simulink model "MATLAB_TEST"  (R2019b)
settings: Solver=FixedStepDiscrete  StartTime=0  StopTime=50  FixedStep=0.0025  RelTol=1e-3
undefined symbols (not defined in the file): BCM_COM_PROC_P20, BCM_COM_PROC_P20_SFW_R2018b, BCM_COM_PROC_P2_5, BCM_COM_PROC_P2_5_SFW_R2018b, BCM_COM_PROC_P5, BCM_COM_PROC_P5_SFW_R2018b, BCMA_ACCU_PT_Conf_Flt, BCMA_ACCU_PT_Unconf_Flt, BCMA_Antiskid_Off_Sanction, BCMA_Avionics_Conf_Flt, BCMA_BCM_CCDL_Conf_Flt, BCMA_BCM_CCDL_Unconf_Flt, BCMA_BCM_DBCU_INHIBITION_Conf_Flt, BCMA_BCM_DBCU_INHIBITION_Unconf_Flt, BCMA_BCP_ALT_Disp_Sw_Conf_Flt, BCMA_BCP_ALT_Disp_Sw_Unconf_Flt, BCMA_BCP_ALT_SW_ON_CMD_Conf_Flt, BCMA_BCP_ALT_SW_ON_CMD_Unconf_Flt, BCMA_BCP_PARK_OFF_SW_CMD_Conf_Flt, BCMA_BCP_PARK_OFF_SW_CMD_Unconf_Flt, BCMA_CF_BSELV_JCL, BCMA_CF_BSELV_JOP, BCMA_CF_BSELV_OC, BCMA_CF_BSELV_SC, BCMA_CF_LH_SV_JCL, BCMA_CF_LH_SV_JOP, BCMA_CF_LH_SV_OC, BCMA_CF_LH_SV_SC, BCMA_CF_PARK_BRK, BCMA_CF_RESIDUAL_PRESS, BCMA_CF_RH_SV_JCL, BCMA_CF_RH_SV_JOP, BCMA_CF_RH_SV_OC, BCMA_CF_RH_SV_SC, BCMA_CF_SELV_JCL, BCMA_CF_SELV_JOP, BCMA_CF_SELV_OC, BCMA_CF_SELV_SC, BCMA_CF_SV_DRIFT, BCMA_DBCU_ALT_MODE_Conf_Flt, BCMA_DBCU_ALT_MODE_Unconf_Flt, BCMA_DBCU_BRK_ORDER_FAIL_Conf_Flt, BCMA_DBCU_BRK_ORDER_FAIL_Unconf_Flt, BCMA_DBCU_Conf_Flt, BCMA_DBCU_DISPATCH_SW_ON_Conf_Flt, BCMA_DBCU_DISPATCH_SW_ON_Unconf_Flt, BCMA_DBCU_FAILED_Conf_Flt, BCMA_DBCU_FAILED_Unconf_Flt, BCMA_DFCS1_Capsule_Validity, BCMA_DFCS1_Label202_Corrupted, BCMA_DFCS1_Label202_Not_Refreshed, BCMA_DFCS1_Label204_Corrupted, BCMA_DFCS1_Label204_Not_Refreshed, BCMA_DFCS1_Label205_Corrupted, BCMA_DFCS1_Label205_Not_Refreshed, BCMA_DFCS1_Label206_Corrupted, BCMA_DFCS1_Label206_Not_Refreshed, BCMA_DFCS1_Label207_Corrupted, BCMA_DFCS1_Label207_Not_Refreshed, BCMA_DFCS3_Capsule_Validity ... (+762)
libraries: simulink x73, lib_MBD_Control x5
(part 9 of 16)

== system MATLAB_TEST/AVIONICS/Brake_Control_Module_Side_A/BCSA Controller CP/DFCSB_Label202_Validity1 ==
  Capsule_Validity : Inport
  Label202_Not_Refreshed : Inport  Port=2
  Label202_Corrupted : Inport  Port=3
  Label202_SSM : Inport  Port=4
  DFCSB_LH_Braking_Cmd : Inport  Port=5
  DFCSB_RH_Braking_Cmd : Inport  Port=6
  Compare To Constant : simulink/Logic and Bit Operations/Compare To Constant  relop=~=  const=3.0  OutDataTypeStr=boolean
  Compare To Constant1 : simulink/Logic and Bit Operations/Compare To Constant  relop=<  const=0  OutDataTypeStr=boolean
  Compare To Constant2 : simulink/Logic and Bit Operations/Compare To Constant  relop=>  const=100  OutDataTypeStr=boolean
  Compare To Constant3 : simulink/Logic and Bit Operations/Compare To Constant  relop=<  const=0  OutDataTypeStr=boolean
  Compare To Constant4 : simulink/Logic and Bit Operations/Compare To Constant  relop=>  const=100  OutDataTypeStr=boolean
  Compare To Zero : simulink/Logic and Bit Operations/Compare To Zero  relop===  OutDataTypeStr=boolean
  Logical Operator : Logic  Operator=OR  Inputs=4  AllPortsSameDT=off  OutDataTypeStr=boolean
  Logical Operator{1..4} (4 alike) : Logic  Operator=OR  AllPortsSameDT=off  OutDataTypeStr=boolean
  Logical Operator5 : Logic  Operator=NOT  AllPortsSameDT=off  OutDataTypeStr=boolean
  Logical Operator6 : Logic  Operator=NOT  AllPortsSameDT=off  OutDataTypeStr=boolean
  LH_Braking_Cmd_Val : Outport  VectorParamsAs1DForOutWhenUnconnected=off
  RH_Braking_Cmd_Val : Outport  Port=2  VectorParamsAs1DForOutWhenUnconnected=off
  wires:
  Logical Operator4/1 -> Logical Operator6/1
  Logical Operator3/1 -> Logical Operator4/2
  Compare To Constant4/1 -> Logical Operator3/1
  Compare To Constant3/1 -> Logical Operator3/2
  Logical Operator2/1 -> Logical Operator5/1
  DFCSB_RH_Braking_Cmd/1 -> Compare To Constant3/1, Compare To Constant4/1
  Compare To Constant1/1 -> Logical Operator1/2
  Logical Operator1/1 -> Logical Operator2/1
  Label202_Not_Refreshed/1 -> Logical Operator/2
  Compare To Constant2/1 -> Logical Operator1/1
  DFCSB_LH_Braking_Cmd/1 -> Compare To Constant2/1, Compare To Constant1/1
  Compare To Zero/1 -> Logical Operator/1
  Capsule_Validity/1 -> Compare To Zero/1
  Label202_Corrupted/1 -> Logical Operator/3
  Label202_SSM/1 -> Compare To Constant/1
  Logical Operator/1 -> Logical Operator4/1, Logical Operator2/2
  Compare To Constant/1 -> Logical Operator/4
  Logical Operator5/1 -> LH_Braking_Cmd_Val/1
  Logical Operator6/1 -> RH_Braking_Cmd_Val/1

== system MATLAB_TEST/AVIONICS/Brake_Control_Module_Side_A/BCSA Controller CP/DFCSB_Long_Accel_Comp ==
  Long_Accel : Inport
  Long_Accel_Val : Inport  Port=2
  Compare To Zero : simulink/Logic and Bit Operations/Compare To Zero  relop===  OutDataTypeStr=boolean
  Init: -0.61 : UnitDelay  InitialCondition=double(single(-0.61))  SampleTime=-1  HasFrameUpgradeWarning=on
  Switch : Switch  Criteria=u2 > Threshold
  Long_Accel_out : Outport  VectorParamsAs1DForOutWhenUnconnected=off
  wires:
  Init: -0.61/1 -> Switch/1
  Switch/1 -> Long_Accel_out/1, Init: -0.61/1
  Long_Accel/1 -> Switch/3
  Compare To Zero/1 -> Switch/2
  Long_Accel_Val/1 -> Compare To Zero/1

== system MATLAB_TEST/AVIONICS/Brake_Control_Module_Side_A/BCSA Controller CP/DFCSB_NLG_WOWs_Comp ==
  NLG_WOWs : Inport
  NLG_WOWs_Val : Inport  Port=2
  Compare To Zero : simulink/Logic and Bit Operations/Compare To Zero  relop===  OutDataTypeStr=boolean
  Init: 0 : UnitDelay  SampleTime=-1  HasFrameUpgradeWarning=on
  Switch : Switch  Criteria=u2 > Threshold
  NLG_WOWs_out : Outport  VectorParamsAs1DForOutWhenUnconnected=off
  wires:
  Init: 0/1 -> Switch/1
  Switch/1 -> NLG_WOWs_out/1, Init: 0/1
  NLG_WOWs/1 -> Switch/3
  Compare To Zero/1 -> Switch/2
  NLG_WOWs_Val/1 -> Compare To Zero/1

== system MATLAB_TEST/AVIONICS/Brake_Control_Module_Side_A/BCSA Controller CP/DFCSB_Pitch_Angle_Comp ==
  Pitch_Angle : Inport
  Pitch_Angle_Val : Inport  Port=2
  Compare To Zero : simulink/Logic and Bit Operations/Compare To Zero  relop===  OutDataTypeStr=boolean
  Init: 0 : UnitDelay  SampleTime=-1  HasFrameUpgradeWarning=on
  Switch : Switch  Criteria=u2 > Threshold
  Pitch_Angle_out : Outport  VectorParamsAs1DForOutWhenUnconnected=off
  wires:
  Pitch_Angle_Val/1 -> Compare To Zero/1
  Compare To Zero/1 -> Switch/2
  Pitch_Angle/1 -> Switch/3
  Switch/1 -> Init: 0/1, Pitch_Angle_out/1
  Init: 0/1 -> Switch/1

== system MATLAB_TEST/AVIONICS/Brake_Control_Module_Side_A/BCSA Controller CP/DFCSB_RH_Braking_Cmd_Comp ==
  Braking_Cmd : Inport
  Braking_Cmd_Val : Inport  Port=2
  Compare To Zero : simulink/Logic and Bit Operations/Compare To Zero  relop===  OutDataTypeStr=boolean
  Init: 0 : UnitDelay  SampleTime=-1  HasFrameUpgradeWarning=on
  Switch : Switch  Criteria=u2 > Threshold
  Braking_Cmd_out : Outport  VectorParamsAs1DForOutWhenUnconnected=off
  wires:
  Braking_Cmd_Val/1 -> Compare To Zero/1
  Compare To Zero/1 -> Switch/2
  Braking_Cmd/1 -> Switch/3
  Switch/1 -> Init: 0/1, Braking_Cmd_out/1
  Init: 0/1 -> Switch/1

== system MATLAB_TEST/AVIONICS/Brake_Control_Module_Side_A/BCSA Controller CP/DFCSB_RMLG_WOWs_Comp ==
  RMLG_WOWs : Inport
  RMLG_WOWs_Val : Inport  Port=2
  Compare To Zero : simulink/Logic and Bit Operations/Compare To Zero  relop===  OutDataTypeStr=boolean
  Init: 0 : UnitDelay  SampleTime=-1  HasFrameUpgradeWarning=on
  Switch : Switch  Criteria=u2 > Threshold
  RMLG_WOWs_out : Outport  VectorParamsAs1DForOutWhenUnconnected=off
  wires:
  RMLG_WOWs_Val/1 -> Compare To Zero/1
  Compare To Zero/1 -> Switch/2
  RMLG_WOWs/1 -> Switch/3
  Switch/1 -> Init: 0/1, RMLG_WOWs_out/1
  Init: 0/1 -> Switch/1

== system MATLAB_TEST/AVIONICS/Brake_Control_Module_Side_A/BCSA Controller CP/DFCSB_TLA_Above_Idle_Comp ==
  TLA_Above_Idle : Inport
  TLA_Above_Idle_Val : Inport  Port=2
  Compare To Zero : simulink/Logic and Bit Operations/Compare To Zero  relop===  OutDataTypeStr=boolean
  Init: 0 : UnitDelay  SampleTime=-1  HasFrameUpgradeWarning=on
  Switch : Switch  Criteria=u2 > Threshold
  TLA_Above_Idle_out : Outport  VectorParamsAs1DForOutWhenUnconnected=off
  wires:
  Init: 0/1 -> Switch/1
  Switch/1 -> TLA_Above_Idle_out/1, Init: 0/1
  TLA_Above_Idle/1 -> Switch/3
  Compare To Zero/1 -> Switch/2
  TLA_Above_Idle_Val/1 -> Compare To Zero/1

== system MATLAB_TEST/AVIONICS/Brake_Control_Module_Side_A/BCSA Controller CP/DFCSB_WOWs_Val_Comp ==
  WOWs_Val_Acq : Inport
  WOWs_Val_Val : Inport  Port=2
  Compare To Zero : simulink/Logic and Bit Operations/Compare To Zero  relop===  OutDataTypeStr=boolean
  Init: 0 : UnitDelay  SampleTime=-1  HasFrameUpgradeWarning=on
  Switch : Switch  Criteria=u2 > Threshold
  WOWs_Val_Acq_out : Outport  VectorParamsAs1DForOutWhenUnconnected=off
  wires:
  Init: 0/1 -> Switch/1
  Switch/1 -> WOWs_Val_Acq_out/1, Init: 0/1
  WOWs_Val_Acq/1 -> Switch/3
  Compare To Zero/1 -> Switch/2
  WOWs_Val_Val/1 -> Compare To Zero/1

== system MATLAB_TEST/AVIONICS/Brake_Control_Module_Side_A/BCSA Controller CP/GenIO_Label021_Validity ==
  Label021_Not_Refreshed : Inport
  Label021_Corrupted : Inport  Port=2
  Label021_SSM : Inport  Port=3
  Hyd_B_Press : Inport  Port=4
  Compare To Constant : simulink/Logic and Bit Operations/Compare To Constant  relop=~=  const=3.0  OutDataTypeStr=boolean
  Compare To Constant1 : simulink/Logic and Bit Operations/Compare To Constant  relop=<  const=0  OutDataTypeStr=boolean
  Compare To Constant2 : simulink/Logic and Bit Operations/Compare To Constant  relop=>  const=5110  OutDataTypeStr=boolean
  Logical Operator : Logic  Operator=OR  Inputs=5  AllPortsSameDT=off  OutDataTypeStr=boolean
  Logical Operator5 : Logic  Operator=NOT  AllPortsSameDT=off  OutDataTypeStr=boolean
  Hyd_B_Press_Val : Outport  VectorParamsAs1DForOutWhenUnconnected=off
  wires:
  Compare To Constant/1 -> Logical Operator/3
  Label021_Corrupted/1 -> Logical Operator/2
  Label021_SSM/1 -> Compare To Constant/1
  Label021_Not_Refreshed/1 -> Logical Operator/1
  Hyd_B_Press/1 -> Compare To Constant2/1, Compare To Constant1/1
  Compare To Constant1/1 -> Logical Operator/4
  Compare To Constant2/1 -> Logical Operator/5
  Logical Operator5/1 -> Hyd_B_Press_Val/1
  Logical Operator/1 -> Logical Operator5/1

== system MATLAB_TEST/AVIONICS/Brake_Control_Module_Side_A/BCSA Controller CP/GenIO_Label022_Validity ==
  Label022_Not_Refreshed : Inport
  Label022_Corrupted : Inport  Port=2
  Label022_SSM : Inport  Port=3
  Hyd_A_Press : Inport  Port=4
  Compare To Constant : simulink/Logic and Bit Operations/Compare To Constant  relop=~=  const=3.0  OutDataTypeStr=boolean
  Compare To Constant1 : simulink/Logic and Bit Operations/Compare To Constant  relop=<  const=0  OutDataTypeStr=boolean
  Compare To Constant2 : simulink/Logic and Bit Operations/Compare To Constant  relop=>  const=5110  OutDataTypeStr=boolean
  Logical Operator1 : Logic  Operator=OR  Inputs=5  AllPortsSameDT=off  OutDataTypeStr=boolean
  Logical Operator5 : Logic  Operator=NOT  AllPortsSameDT=off  OutDataTypeStr=boolean
  Hyd_A_Press_Val : Outport  VectorParamsAs1DForOutWhenUnconnected=off
  wires:
  Label022_Not_Refreshed/1 -> Logical Operator1/1
  Label022_SSM/1 -> Compare To Constant/1
  Label022_Corrupted/1 -> Logical Operator1/2
  Compare To Constant/1 -> Logical Operator1/3
  Hyd_A_Press/1 -> Compare To Constant2/1, Compare To Constant1/1
  Compare To Constant1/1 -> Logical Operator1/4
  Compare To Constant2/1 -> Logical Operator1/5
  Logical Operator5/1 -> Hyd_A_Press_Val/1
  Logical Operator1/1 -> Logical Operator5/1

== system MATLAB_TEST/AVIONICS/Brake_Control_Module_Side_A/BCSA Controller CP/GenIO_Label272_Validity ==
  Label272_Not_Refreshed : Inport
  Label272_Corrupted : Inport  Port=2
  Label272_SSM : Inport  Port=3
  Compare To Constant : simulink/Logic and Bit Operations/Compare To Constant  relop=~=  const=3.0  OutDataTypeStr=boolean
  Logical Operator : Logic  Operator=OR  Inputs=3  AllPortsSameDT=off  OutDataTypeStr=boolean
  Logical Operator5 : Logic  Operator=NOT  AllPortsSameDT=off  OutDataTypeStr=boolean
  Engine1_Running_Val : Outport  VectorParamsAs1DForOutWhenUnconnected=off
  wires:
  Label272_Not_Refreshed/1 -> Logical Operator/1
  Label272_SSM/1 -> Compare To Constant/1
  Label272_Corrupted/1 -> Logical Operator/2
  Compare To Constant/1 -> Logical Operator/3
  Logical Operator5/1 -> Engine1_Running_Val/1
  Logical Operator/1 -> Logical Operator5/1

== system MATLAB_TEST/AVIONICS/Brake_Control_Module_Side_A/BCSA Controller CP/GenIO_Label273_Validity ==
  Label273_Not_Refreshed : Inport
  Label273_Corrupted : Inport  Port=2
  Label273_SSM : Inport  Port=3
  Compare To Constant : simulink/Logic and Bit Operations/Compare To Constant  relop=~=  const=3.0  OutDataTypeStr=boolean
  Logical Operator : Logic  Operator=OR  Inputs=3  AllPortsSameDT=off  OutDataTypeStr=boolean
  Logical Operator5 : Logic  Operator=NOT  AllPortsSameDT=off  OutDataTypeStr=boolean
  Engine2_Running_Val : Outport  VectorParamsAs1DForOutWhenUnconnected=off
  wires:
  Compare To Constant/1 -> Logical Operator/3
  Label273_Corrupted/1 -> Logical Operator/2
  Label273_SSM/1 -> Compare To Constant/1
  Label273_Not_Refreshed/1 -> Logical Operator/1
  Logical Operator5/1 -> Engine2_Running_Val/1
  Logical Operator/1 -> Logical Operator5/1

== system MATLAB_TEST/AVIONICS/Brake_Control_Module_Side_A/BCSA Controller CP/Inadvertent Braking Order BSELV Failure Mode ==
  SELV_High_Side_Cmd_Order : Inport
  CP_Inadvertent_Braking_Order_BSELV_DBSMA : Inport  Port=2  SampleTime=0.02
  Constant1 : Constant  SampleTime=0.02
  Switch1 : Switch  Criteria=u2 > Threshold
  HASELV_CMD : Outport  VectorParamsAs1DForOutWhenUnconnected=off
  wires:
  Constant1/1 -> Switch1/1
  SELV_High_Side_Cmd_Order/1 -> Switch1/3
  Switch1/1 -> HASELV_CMD/1
  CP_Inadvertent_Braking_Order_BSELV_DBSMA/1 -> Switch1/2

== system MATLAB_TEST/AVIONICS/Brake_Control_Module_Side_A/BCSA Controller CP/Inadvertent Braking Order DBSMA Failure Mode ==
  LH_HASV_CURRENT_in : Inport
  RH_HASV_CURRENT_in : Inport  Port=2
  CP_Inadvertent_Braking_Order_BSELV_DBSMA : Inport  Port=3  SampleTime=0.005
  CP_Erroneous_Current_To_LH : Inport  Port=4  SampleTime=0.005
  CP_Erroneous_Current_To_RH : Inport  Port=5  SampleTime=0.005
  Constant1 : Constant  Value=40  SampleTime=0.005
  Constant2 : Constant  Value=40  SampleTime=0.005
  Logical Operator : Logic  Operator=OR  AllPortsSameDT=off  OutDataTypeStr=boolean
  Logical Operator1 : Logic  Operator=OR  AllPortsSameDT=off  OutDataTypeStr=boolean
  Switch1 : Switch  Criteria=u2 > Threshold
  Switch2 : Switch  Criteria=u2 > Threshold
  LH_HASV_CURRENT : Outport  VectorParamsAs1DForOutWhenUnconnected=off
  RH_HASV_CURRENT : Outport  Port=2  VectorParamsAs1DForOutWhenUnconnected=off
  wires:
  CP_Inadvertent_Braking_Order_BSELV_DBSMA/1 -> Logical Operator1/1, Logical Operator/2
  Switch1/1 -> LH_HASV_CURRENT/1
  LH_HASV_CURRENT_in/1 -> Switch1/3
  Constant1/1 -> Switch1/1
  Switch2/1 -> RH_HASV_CURRENT/1
  RH_HASV_CURRENT_in/1 -> Switch2/3
  Constant2/1 -> Switch2/1
  Logical Operator/1 -> Switch1/2
  CP_Erroneous_Current_To_LH/1 -> Logical Operator/1
  Logical Operator1/1 -> Switch2/2
  CP_Erroneous_Current_To_RH/1 -> Logical Operator1/2

== system MATLAB_TEST/AVIONICS/Brake_Control_Module_Side_A/BCSA Controller CP/Inadvertent Braking Order Failure Mode ==
  DFCSA_LH_Braking_Cmd_in : Inport
  DFCSA_RH_Braking_Cmd_in : Inport  Port=2
  CP_Inadvertent_Braking_Order_Acquisition : Inport  Port=3
  Constant : Constant  Value=100  SampleTime=-1
  Constant1 : Constant  Value=100  SampleTime=-1
  Switch1 : Switch  Criteria=u2 > Threshold
  Switch2 : Switch  Criteria=u2 > Threshold
  DFCSA_LH_Braking_Cmd : Outport  VectorParamsAs1DForOutWhenUnconnected=off
  DFCSA_RH_Braking_Cmd : Outport  Port=2  VectorParamsAs1DForOutWhenUnconnected=off
  wires:
  DFCSA_RH_Braking_Cmd_in/1 -> Switch2/3
  DFCSA_LH_Braking_Cmd_in/1 -> Switch1/3
  Switch1/1 -> DFCSA_LH_Braking_Cmd/1
  Switch2/1 -> DFCSA_RH_Braking_Cmd/1
  CP_Inadvertent_Braking_Order_Acquisition/1 -> Switch2/2, Switch1/2
  Constant/1 -> Switch1/1
  Constant1/1 -> Switch2/1

== system MATLAB_TEST/AVIONICS/Brake_Control_Module_Side_A/BCSA Controller CP/Left Inner Wheel Speed Emission Failure Mode ==
  note: Wheel speed order:
      | 1) Left outer
      | 2) Left inner
      | 3) Right inner
      | 4) Right outer
  LHI_Wheel_Speed_in : Inport
  Wheel_Speed_2_Erroneous_Emission : Inport  Port=2  SampleTime=0.0025
  Constant1 : Constant  Value=BCMA_WheelSpeed2_Erroneous_Emission_Value  OutDataTypeStr=single  SampleTime=0.0025
  Switch1 : Switch  Criteria=u2 > Threshold
  LHI_Wheel_Speed : Outport  VectorParamsAs1DForOutWhenUnconnected=off
  wires:
  Wheel_Speed_2_Erroneous_Emission/1 -> Switch1/2
  Switch1/1 -> LHI_Wheel_Speed/1
  LHI_Wheel_Speed_in/1 -> Switch1/3
  Constant1/1 -> Switch1/1

== system MATLAB_TEST/AVIONICS/Brake_Control_Module_Side_A/BCSA Controller CP/Left Inner Wheel Speed Failure Modes ==
  note: Wheel speed order:
      | 1) Left outer
      | 2) Left inner
      | 3) Right inner
      | 4) Right outer
  LH_IN_WHEEL_SPEED_in : Inport
  Wheel_Speed_2_Erroneous_Acquisition : Inport  Port=2
  Wheel_Speed_2_Loss : Inport  Port=3
  AIG3 : lib_MBD_Control/Logics/Signal Routing/AIG3  Tag=AIG4
      settings: SourceProductName=MBD
  Constant : Constant  SampleTime=-1
  Constant1 : Constant  Value=BCMA_WheelSpeed2_Erroneous_Acq_Value  SampleTime=-1
  LH_IN_WHEEL_SPEED : Outport  VectorParamsAs1DForOutWhenUnconnected=off
  wires:
  LH_IN_WHEEL_SPEED_in/1 -> AIG3/5
  AIG3/1 -> LH_IN_WHEEL_SPEED/1
  Wheel_Speed_2_Erroneous_Acquisition/1 -> AIG3/1
  Wheel_Speed_2_Loss/1 -> AIG3/2
  Constant/1 -> AIG3/4
  Constant1/1 -> AIG3/3

== system MATLAB_TEST/AVIONICS/Brake_Control_Module_Side_A/BCSA Controller CP/Left Outer Wheel Speed Emission Failure Mode ==
  note: Wheel speed order:
      | 1) Left outer
      | 2) Left inner
      | 3) Right inner
      | 4) Right outer
  LHO_Wheel_Speed_in : Inport
  Wheel_Speed_1_Erroneous_Emission : Inport  Port=2  SampleTime=0.0025
  Constant1 : Constant  Value=BCMA_WheelSpeed1_Erroneous_Emission_Value  OutDataTypeStr=single  SampleTime=0.0025
  Switch1 : Switch  Criteria=u2 > Threshold
  LHO_Wheel_Speed : Outport  VectorParamsAs1DForOutWhenUnconnected=off
  wires:
  Constant1/1 -> Switch1/1
  LHO_Wheel_Speed_in/1 -> Switch1/3
  Switch1/1 -> LHO_Wheel_Speed/1
  Wheel_Speed_1_Erroneous_Emission/1 -> Switch1/2

== system MATLAB_TEST/AVIONICS/Brake_Control_Module_Side_A/BCSA Controller CP/Left Outer Wheel Speed Failure Modes ==
  note: Wheel speed order:
      | 1) Left outer
      | 2) Left inner
      | 3) Right inner
      | 4) Right outer
  LH_OUT_WHEEL_SPEED_in : Inport
  Wheel_Speed_1_Erroneous_Acquisition : Inport  Port=2
  Wheel_Speed_1_Loss : Inport  Port=3
  AIG3 : lib_MBD_Control/Logics/Signal Routing/AIG3  Tag=AIG4
      settings: SourceProductName=MBD
  Constant : Constant  SampleTime=-1
  Constant1 : Constant  Value=BCMA_WheelSpeed1_Erroneous_Acq_Value  SampleTime=-1
  LH_OUT_WHEEL_SPEED : Outport  VectorParamsAs1DForOutWhenUnconnected=off
  wires:
  Constant1/1 -> AIG3/3
  Constant/1 -> AIG3/4
  Wheel_Speed_1_Loss/1 -> AIG3/2
  Wheel_Speed_1_Erroneous_Acquisition/1 -> AIG3/1
  AIG3/1 -> LH_OUT_WHEEL_SPEED/1
  LH_OUT_WHEEL_SPEED_in/1 -> AIG3/5

== system MATLAB_TEST/AVIONICS/Brake_Control_Module_Side_A/BCSA Controller CP/Left Pressure Transducer Failure Mode ==
  LH_PT_PRESSURE_in : Inport
  LH_PT_Erroneous_Acquisition : Inport  Port=2
  Constant1 : Constant  Value=BCMA_LHPT_Erroneous_Value  SampleTime=-1
  Switch1 : Switch  Criteria=u2 > Threshold
  LH_PT_PRESSURE : Outport  VectorParamsAs1DForOutWhenUnconnected=off
  wires:
  LH_PT_Erroneous_Acquisition/1 -> Switch1/2
  Switch1/1 -> LH_PT_PRESSURE/1
  LH_PT_PRESSURE_in/1 -> Switch1/3
  Constant1/1 -> Switch1/1

== system MATLAB_TEST/AVIONICS/Brake_Control_Module_Side_A/BCSA Controller CP/Right Inner Wheel Speed Emission Failure Mode ==
  note: Wheel speed order:
      | 1) Left outer
      | 2) Left inner
      | 3) Right inner
      | 4) Right outer
  RHI_Wheel_Speed_in : Inport
  Wheel_Speed_3_Erroneous_Emission : Inport  Port=2  SampleTime=0.0025
  Constant1 : Constant  Value=BCMA_WheelSpeed3_Erroneous_Emission_Value  OutDataTypeStr=single  SampleTime=0.0025
  Switch1 : Switch  Criteria=u2 > Threshold
  RHI_Wheel_Speed : Outport  VectorParamsAs1DForOutWhenUnconnected=off
  wires:
  Constant1/1 -> Switch1/1
  RHI_Wheel_Speed_in/1 -> Switch1/3
  Switch1/1 -> RHI_Wheel_Speed/1
  Wheel_Speed_3_Erroneous_Emission/1 -> Switch1/2

== system MATLAB_TEST/AVIONICS/Brake_Control_Module_Side_A/BCSA Controller CP/Right Inner Wheel Speed Failure Modes ==
  note: Wheel speed order:
      | 1) Left outer
      | 2) Left inner
      | 3) Right inner
      | 4) Right outer
  RH_IN_WHEEL_SPEED_in : Inport
  Wheel_Speed_3_Erroneous_Acquisition : Inport  Port=2
  Wheel_Speed_3_Loss : Inport  Port=3
  AIG3 : lib_MBD_Control/Logics/Signal Routing/AIG3  Tag=AIG4
      settings: SourceProductName=MBD
  Constant : Constant  SampleTime=-1
  Constant1 : Constant  Value=BCMA_WheelSpeed3_Erroneous_Acq_Value  SampleTime=-1
  RH_IN_WHEEL_SPEED : Outport  VectorParamsAs1DForOutWhenUnconnected=off
  wires:
  RH_IN_WHEEL_SPEED_in/1 -> AIG3/5
  AIG3/1 -> RH_IN_WHEEL_SPEED/1
  Wheel_Speed_3_Erroneous_Acquisition/1 -> AIG3/1
  Wheel_Speed_3_Loss/1 -> AIG3/2
  Constant/1 -> AIG3/4
  Constant1/1 -> AIG3/3

== system MATLAB_TEST/AVIONICS/Brake_Control_Module_Side_A/BCSA Controller CP/Right Outer Wheel Speed Emission Failure Mode ==
  note: Wheel speed order:
      | 1) Left outer
      | 2) Left inner
      | 3) Right inner
      | 4) Right outer
  RHO_Wheel_Speed_in : Inport
  Wheel_Speed_4_Erroneous_Emission : Inport  Port=2  SampleTime=0.0025
  Constant1 : Constant  Value=BCMA_WheelSpeed4_Erroneous_Emission_Value  OutDataTypeStr=single  SampleTime=0.0025
  Switch1 : Switch  Criteria=u2 > Threshold
  RHO_Wheel_Speed : Outport  VectorParamsAs1DForOutWhenUnconnected=off
  wires:
  Wheel_Speed_4_Erroneous_Emission/1 -> Switch1/2
  Switch1/1 -> RHO_Wheel_Speed/1
  RHO_Wheel_Speed_in/1 -> Switch1/3
  Constant1/1 -> Switch1/1

== system MATLAB_TEST/AVIONICS/Brake_Control_Module_Side_A/BCSA Controller CP/Right Outer Wheel Speed Failure Modes ==
  note: Wheel speed order:
      | 1) Left outer
      | 2) Left inner
      | 3) Right inner
      | 4) Right outer
  RH_OUT_WHEEL_SPEED_in : Inport
  Wheel_Speed_4_Erroneous_Acquisition : Inport  Port=2
  Wheel_Speed_4_Loss : Inport  Port=3
  AIG3 : lib_MBD_Control/Logics/Signal Routing/AIG3  Tag=AIG4
      settings: SourceProductName=MBD
  Constant : Constant  SampleTime=-1
  Constant1 : Constant  Value=BCMA_WheelSpeed4_Erroneous_Acq_Value  SampleTime=-1
  RH_OUT_WHEEL_SPEED : Outport  VectorParamsAs1DForOutWhenUnconnected=off
  wires:
  Constant1/1 -> AIG3/3
  Constant/1 -> AIG3/4
  Wheel_Speed_4_Loss/1 -> AIG3/2
  Wheel_Speed_4_Erroneous_Acquisition/1 -> AIG3/1
  AIG3/1 -> RH_OUT_WHEEL_SPEED/1
  RH_OUT_WHEEL_SPEED_in/1 -> AIG3/5

== system MATLAB_TEST/AVIONICS/Brake_Control_Module_Side_A/BCSA Controller CP/Right Pressure Transducer Failure Mode ==
  RH_PT_PRESSURE_in : Inport
  RH_PT_Erroneous_Acquisition : Inport  Port=2
  Constant1 : Constant  Value=BCMA_RHPT_Erroneous_Value  SampleTime=-1
  Switch1 : Switch  Criteria=u2 > Threshold
  RH_PT_PRESSURE : Outport  VectorParamsAs1DForOutWhenUnconnected=off
  wires:
  Constant1/1 -> Switch1/1
  RH_PT_PRESSURE_in/1 -> Switch1/3
  Switch1/1 -> RH_PT_PRESSURE/1
  RH_PT_Erroneous_Acquisition/1 -> Switch1/2

== system MATLAB_TEST/AVIONICS/Brake_Control_Module_Side_A/BCSA Controller CP/Tuning Management ==
  note: Not used
  FTI_switch_1 : Inport
  FTI_switch_2 : Inport  Port=2
  FTI_switch_3 : Inport  Port=3
  FTI_switch_4 : Inport  Port=4
  FTI_switch_5 : Inport  Port=5
  BCM_Config : Inport  Port=6
  Conf1 : Subsystem
  Conf2 : Subsystem
  Conf3 : Subsystem
  Multiport Switch : MultiPortSwitch  DataPortOrder=Zero-based contiguous  zeroidx=on
  Terminator{29..33} (5 alike) : Terminator
  BCM_Tuning : Outport  VectorParamsAs1DForOutWhenUnconnected=off
  wires:
  FTI_switch_2/1 -> Terminator30/1
  FTI_switch_4/1 -> Terminator32/1
  FTI_switch_3/1 -> Terminator31/1
  FTI_switch_1/1 -> Terminator29/1
  FTI_switch_5/1 -> Terminator33/1
  Multiport Switch/1 -> BCM_Tuning/1
  BCM_Config/1 -> Multiport Switch/1
  Conf1/1(Out1) -> Multiport Switch/2
  Conf2/1(Out1) -> Multiport Switch/3
  Conf3/1(Out1) -> Multiport Switch/4
